simulink model "Simulation"  (R2022b)
settings: Solver=FixedStepAuto  StartTime=0.0  StopTime=20  FixedStep=1e-2  RelTol=1e-3
undefined symbols (not defined in the file): A, B, C, D, Gain, initial_conditions
settings Model: Creator=fades  LastModifiedBy=fades

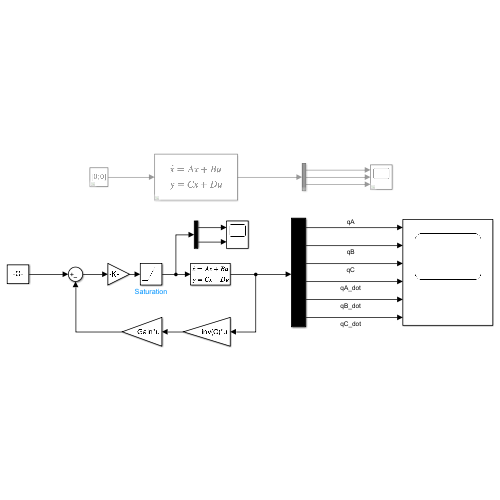
[thumbnail: Simulink's stored preview of the top-level diagram]
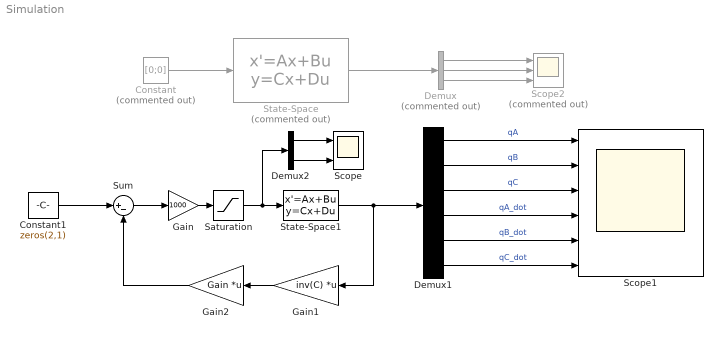
== system Simulation ==
  Constant : Constant  Commented=on  Value=[0;0]
  Constant1 : Constant  Value=zeros(2,1)
  Demux : Demux  Commented=on  Outputs=3
  Demux1 : Demux  Outputs=6
  Demux2 : Demux  Outputs=2
  Gain : Gain  Gain=1000
  Gain1 : Gain  Gain=inv(C)  Multiplication=Matrix(K*u)
  Gain2 : Gain  Gain=Gain  Multiplication=Matrix(K*u)
  Saturation : Saturate  UpperLimit=120  LowerLimit=-120
  Scope : Scope  NumInputPorts=2
  Scope1 : Scope  NumInputPorts=6
  Scope2 : Scope  Commented=on  NumInputPorts=3
  State-Space : StateSpace  Commented=on  A=A  B=B  C=C  D=D  InitialCondition=initial_conditions
  State-Space1 : StateSpace  A=A  B=B  C=C  D=D  InitialCondition=initial_conditions
  Sum : Sum  Inputs=|+-
  wires:
  Demux/3 -> Scope2/3
  Demux/2 -> Scope2/2
  Demux/1 -> Scope2/1
  State-Space/1 -> Demux/1
  Constant/1 -> State-Space/1
  State-Space1/1 -> Gain1/1, Demux1/1
  Demux1/2 -> Scope1/2  "qB"
  Demux1/3 -> Scope1/3  "qC"
  Demux1/1 -> Scope1/1  "qA"
  Demux1/4 -> Scope1/4  "qA_dot"
  Demux1/5 -> Scope1/5  "qB_dot"
  Demux1/6 -> Scope1/6  "qC_dot"
  Constant1/1 -> Sum/1
  Saturation/1 -> Demux2/1, State-Space1/1
  Gain1/1 -> Gain2/1
  Gain2/1 -> Sum/2
  Sum/1 -> Gain/1
  Gain/1 -> Saturation/1
  Demux2/1 -> Scope/1
  Demux2/2 -> Scope/2
